simulink model "zadatak2a"  (R2023b)
settings: Solver=VariableStepAuto  StartTime=0.0  StopTime=100  RelTol=1e-3
settings Model: Creator=lvuke  LastModifiedBy=lvuke

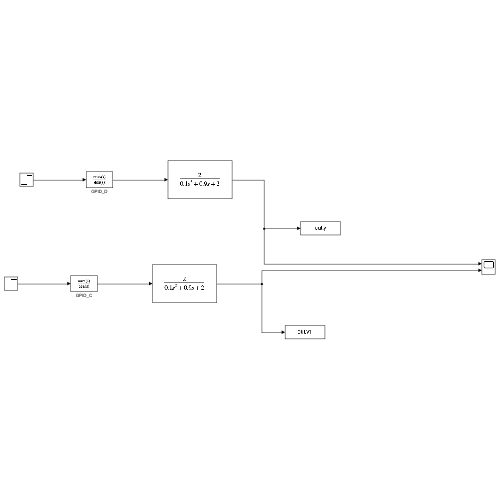
[thumbnail: Simulink's stored preview of the top-level diagram]
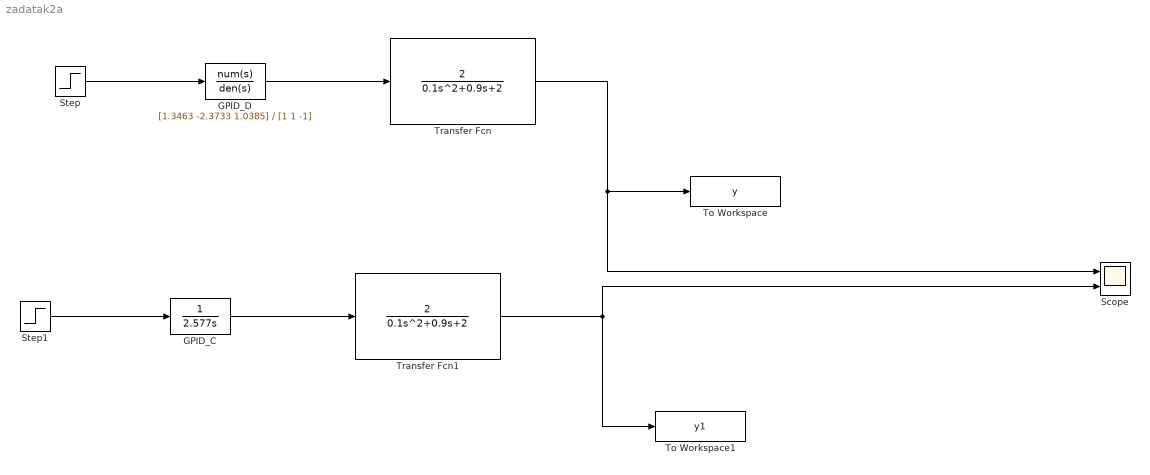
== system zadatak2a ==
  GPID_C : TransferFcn  Numerator=[0 0 1]  Denominator=[0 2.577 0]
  GPID_D : TransferFcn  Numerator=[1.3463 -2.3733 1.0385]  Denominator=[1 1 -1]
  Scope : Scope  NumInputPorts=2
  Step : Step  Time=0  After=3  SampleTime=0
  Step1 : Step  Time=0  After=3  SampleTime=0
  To Workspace : ToWorkspace  VariableName=y  SaveFormat=Timeseries  SampleTime=-1
  To Workspace1 : ToWorkspace  VariableName=y1  SaveFormat=Timeseries  SampleTime=-1
  Transfer Fcn : TransferFcn  Numerator=[2]  Denominator=[0.1 0.9 2]
  Transfer Fcn1 : TransferFcn  Numerator=[2]  Denominator=[0.1 0.9 2]
  wires:
  Transfer Fcn/1 -> To Workspace/1, Scope/1
  Step/1 -> GPID_D/1
  GPID_D/1 -> Transfer Fcn/1
  GPID_C/1 -> Transfer Fcn1/1
  Transfer Fcn1/1 -> To Workspace1/1, Scope/2
  Step1/1 -> GPID_C/1
